simulink model "active_suspension_sim"  (R2021a)
settings: Solver=ode45  StartTime=0.0  StopTime=10.0  RelTol=1e-3
values from neighbouring files (symbols this model uses):
  A = [[0 1 0 0 0];[-(cw+cs)/mw -ds/mw cs/mw ds/mw -1/mw];[0 0 0 1 0];[cs/mc ds/mc -cs/mc -ds/mc 1/mc];[0 0 0 0 -1/tau]]    [active_suspension_ctrl_design.m]
  B1 = [B H]    [active_suspension_ctrl_design.m]
  C = [[-1 0 1 0 0];[cs/mc ds/mc -cs/mc -ds/mc 1/mc]]    [active_suspension_ctrl_design.m]
  C1 = eye(5)    [active_suspension_ctrl_design.m]
  D1 = zeros(5,2)    [active_suspension_ctrl_design.m]
undefined symbols (not defined in the file or in its folder): K
settings Model: Creator=JonasMac  LastModifiedBy=ThnkPad
settings SolverCC: AlgebraicLoopSolver=TrustRegion
settings DataIOCC: LimitDataPoints=on  SaveFormat=Array  SignalLoggingSaveFormat=ModelDataLogs  ReturnWorkspaceOutputs=off
settings OptimizationCC: BlockReduction=off  BooleanDataType=off  LifeSpan=inf
settings DebuggingCC: SaveWithParameterizedLinksMsg=none  UnderspecifiedInitializationDetection=Classic  MergeDetectMultiDrivingBlocksExec=none  SignalResolutionControl=TryResolveAllWithWarning  MultiTaskDSMMsg=warning  MultiTaskCondExecSysMsg=none  SFUnexpectedBacktrackingDiag=warning  SFNoUnconditionalDefaultTransitionDiag=warning  SFExecutionAtInitializationDiag=none  SFMachineParentedDataDiag=warning  ArithmeticOperatorsInVariantConditions=warning
settings HardwareCC: ProdBitPerPointer=32  ProdBitPerSizeT=32  ProdBitPerPtrDiffT=32  ProdLargestAtomicFloat=None  ProdIntDivRoundTo=Undefined  ProdEndianess=Unspecified  ProdWordSize=32  ProdHWDeviceType=32-bit Generic  TargetUnknown=on
settings ModelReferenceCC: PropagateSignalLabelsOutOfModel=off
settings SFSimCC: SimUseLocalCustomCode=off  CustomCodeUndefinedFunction=UseInterfaceOnly
settings RTWCC: RTWUseLocalCustomCode=off
settings CodeAppCC: StateflowObjectComments=on
settings GRTTargetCC: TargetLangStandard=C89/C90 (ANSI)
settings ConfigComp: CovMetricSettings=dw  CovSaveCumulativeToWorkspaceVar=on  CovSaveSingleToWorkspaceVar=on  CovExternalEMLEnable=off

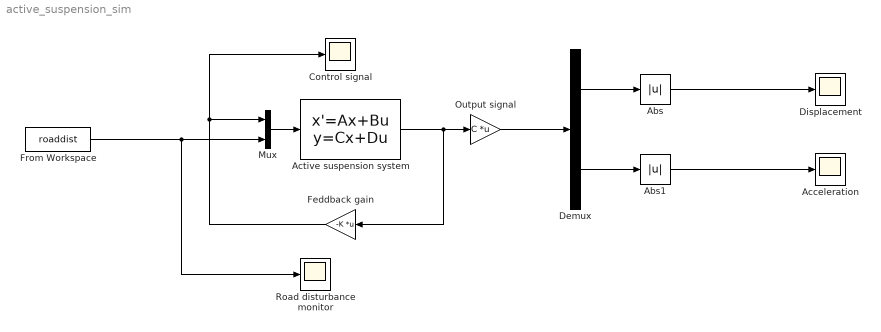
== system active_suspension_sim ==
  Abs : Abs
  Abs1 : Abs
  Acceleration : Scope
  Active suspension system : StateSpace  A=A  B=B1  C=C1  D=D1
  Control signal : Scope
  Demux : Demux  Outputs=2
  Displacement : Scope
  Feddback gain : Gain  Gain=-K  Multiplication=Matrix(K*u)
  From Workspace : FromWorkspace  VariableName=roaddist
  Mux : Mux  Inputs=2
  Output signal : Gain  Gain=C  Multiplication=Matrix(K*u)
  Road disturbance monitor : Scope
  wires:
  Demux/1 -> Abs/1
  Active suspension system/1 -> Feddback gain/1, Output signal/1
  Feddback gain/1 -> Mux/1, Control signal/1
  Mux/1 -> Active suspension system/1
  Output signal/1 -> Demux/1
  Demux/2 -> Abs1/1
  From Workspace/1 -> Road disturbance monitor/1, Mux/2
  Abs/1 -> Displacement/1
  Abs1/1 -> Acceleration/1
